simulink model "mdl4_20160413_004644"  (R2014a)
settings: Solver=FixedStepDiscrete  SolverMode=SingleTasking  StartTime=TIME(1)  StopTime=TIME(end)  FixedStep=SIMSTEP  RelTol=1e-3
model workspace (MAT data in the model file):
  autoc_mdd_data01 : struct (value not decoded)
undefined symbols (not defined in the file): Parameter113, Parameter131, Parameter132, Parameter144, Parameter51, Parameter52, Parameter53, Parameter54, Parameter69, Parameter91, SIMSTEP
(part 3 of 3)

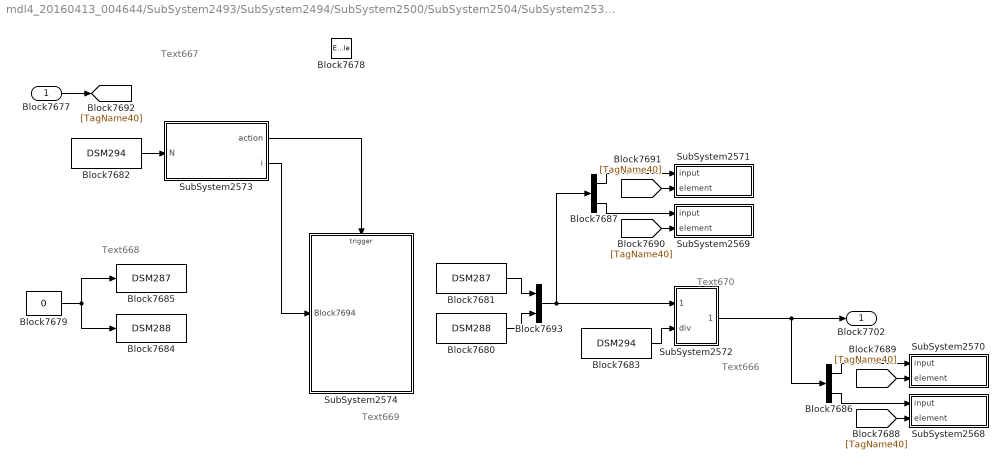
== system mdl4_20160413_004644/SubSystem2493/SubSystem2494/SubSystem2500/SubSystem2504/SubSystem2533/SubSystem2567 ==
  note: Text670
  note: Text669
  note: Text668
  note: Text667
  note: Text666
  Block7677 : Inport
  Block7678 : EnablePort
  Block7679 : Constant  Value=0  OutDataTypeStr=double  SampleTime=-1
  Block7680 : DataStoreRead  Priority=30  DataStoreName=DSM288
      settings: AttributesFormatString=Attribute1963
  Block7681 : DataStoreRead  Priority=30  DataStoreName=DSM287
      settings: AttributesFormatString=Attribute1964
  Block7682 : DataStoreRead  DataStoreName=DSM294
  Block7683 : DataStoreRead  DataStoreName=DSM294
  Block7684 : DataStoreWrite  Priority=10  DataStoreName=DSM288
      settings: AttributesFormatString=Attribute1965
  Block7685 : DataStoreWrite  Priority=10  DataStoreName=DSM287
      settings: AttributesFormatString=Attribute1966
  Block7686 : Demux  Outputs=2
  Block7687 : Demux  Outputs=2
  Block7693 : Mux  Inputs=2
  SubSystem2568 : Subsystem  TreatAsAtomicUnit=on  mask(***ATC.DSWVEC***){bd_version=1.01.A, r0=DSM290, r1=-1, r2=, r3=, r4=, r5=, r6=, r7=, r8=, r9=, c0=, c1=, c2=, c3=, c4=, c5=, c6=, c7=, c8=, c9=}
      mask prompts: bd_version "Version"
      mask help: これはAutoCからのブロックです．編集禁止．
      settings: OpenFcn=warndlg('変更禁止!');
      mask Help: web(ui_blockhelpmng(gcb));
      mask Display: disp('ATC.DSRVEC')
  SubSystem2569 : Subsystem  TreatAsAtomicUnit=on  mask(***ATC.DSWVEC***){bd_version=1.01.A, r0=DSM292, r1=-1, r2=, r3=, r4=, r5=, r6=, r7=, r8=, r9=, c0=, c1=, c2=, c3=, c4=, c5=, c6=, c7=, c8=, c9=}
      mask prompts: bd_version "Version"
      mask help: これはAutoCからのブロックです．編集禁止．
      settings: OpenFcn=warndlg('変更禁止!');
      mask Help: web(ui_blockhelpmng(gcb));
      mask Display: disp('ATC.DSRVEC')
  SubSystem2570 : Subsystem  TreatAsAtomicUnit=on  mask(***ATC.DSWVEC***){bd_version=1.01.A, r0=DSM289, r1=-1, r2=, r3=, r4=, r5=, r6=, r7=, r8=, r9=, c0=, c1=, c2=, c3=, c4=, c5=, c6=, c7=, c8=, c9=}
      mask prompts: bd_version "Version"
      mask help: これはAutoCからのブロックです．編集禁止．
      settings: OpenFcn=warndlg('変更禁止!');
      mask Help: web(ui_blockhelpmng(gcb));
      mask Display: disp('ATC.DSRVEC')
  SubSystem2571 : Subsystem  TreatAsAtomicUnit=on  mask(***ATC.DSWVEC***){bd_version=1.01.A, r0=DSM291, r1=-1, r2=, r3=, r4=, r5=, r6=, r7=, r8=, r9=, c0=, c1=, c2=, c3=, c4=, c5=, c6=, c7=, c8=, c9=}
      mask prompts: bd_version "Version"
      mask help: これはAutoCからのブロックです．編集禁止．
      settings: OpenFcn=warndlg('変更禁止!');
      mask Help: web(ui_blockhelpmng(gcb));
      mask Display: disp('ATC.DSRVEC')
  SubSystem2572 : Subsystem  TreatAsAtomicUnit=on  mask(***ATC.DIVISION***){bd_version=1.01.A, r0=チェック無し, r1=, r2=, r3=, r4=, r5=, r6=, r7=, r8=, r9=, c0=, c1=, c2=, c3=, c4=, c5=, c6=, c7=, c8=, c9=}
      mask prompts: bd_version "Version"
      mask help: これはAutoCからのブロックです．編集禁止．
      settings: OpenFcn=warndlg('変更禁止!');
      mask Help: web(ui_blockhelpmng(gcb));
  SubSystem2573 : Subsystem  Priority=20  TreatAsAtomicUnit=on  mask(***ATC.ITERATOR***){}
      mask help: これはAutoCからのブロックです．編集禁止．
      settings: AttributesFormatString=Attribute1967  OpenFcn=warndlg('変更禁止!');  RTWSystemCode=Inline
  SubSystem2574 : Subsystem  TreatAsAtomicUnit=on
  Block7702 : Outport
  wires:
  Block7679/1 -> Block7684/1, Block7685/1
  Block7687/2 -> SubSystem2569/1(input)
  [TagName40] -> SubSystem2569/2(element)
  Block7687/1 -> SubSystem2571/1(input)
  [TagName40] -> SubSystem2571/2(element)
  Block7686/2 -> SubSystem2568/1(input)
  [TagName40] -> SubSystem2568/2(element)
  Block7686/1 -> SubSystem2570/1(input)
  [TagName40] -> SubSystem2570/2(element)
  Block7693/1 -> Block7687/1, SubSystem2572/1(mult)
  Block7680/1 -> Block7693/2
  Block7681/1 -> Block7693/1
  SubSystem2572/1(Out) -> Block7686/1, Block7702/1
  Block7683/1 -> SubSystem2572/2(div)
  SubSystem2573/2(i) -> SubSystem2574/1(Block7694)
  SubSystem2573/1(action) -> SubSystem2574/Trigger
  Block7682/1 -> SubSystem2573/1(N)
  Block7677/1 -> [TagName40]

== system mdl4_20160413_004644/SubSystem2493/SubSystem2494/SubSystem2500/SubSystem2504/SubSystem2533/SubSystem2537/SubSystem2538 ==
  note: ***編集禁止***
  input : Inport
  element : Inport  Port=2
  Assignment : Assignment  IndexOptions=Index vector (port)  OutputSizes=[1 1]
  Inside_DSR : DataStoreRead  DataStoreName=DSM293
  Inside_DSW : DataStoreWrite  DataStoreName=DSM293
  wires:
  Assignment/1 -> Inside_DSW/1
  Inside_DSR/1 -> Assignment/1
  input/1 -> Assignment/2
  element/1 -> Assignment/3

== system mdl4_20160413_004644/SubSystem2493/SubSystem2494/SubSystem2500/SubSystem2504/SubSystem2533/SubSystem2537/SubSystem2539 ==
  note: ***編集禁止***
  input : Inport
  element : Inport  Port=2
  Assignment : Assignment  IndexOptions=Index vector (port)  OutputSizes=[1 1]
  Inside_DSR : DataStoreRead  DataStoreName=DSM295
  Inside_DSW : DataStoreWrite  DataStoreName=DSM295
  wires:
  Assignment/1 -> Inside_DSW/1
  Inside_DSR/1 -> Assignment/1
  input/1 -> Assignment/2
  element/1 -> Assignment/3

== system mdl4_20160413_004644/SubSystem2493/SubSystem2494/SubSystem2500/SubSystem2504/SubSystem2533/SubSystem2537/SubSystem2540 ==
  note: ***編集禁止***
  In1 : Inport
  In2 : Inport  Port=2
  RO1 : RelationalOperator  Operator===  InputSameDT=on
  single1 : DataTypeConversion  OutDataTypeStr=single  SaturateOnIntegerOverflow=on  RndMeth=Zero
  single2 : DataTypeConversion  OutDataTypeStr=single  SaturateOnIntegerOverflow=on  RndMeth=Zero
  Out1 : Outport
  wires:
  single2/1 -> RO1/2
  single1/1 -> RO1/1
  In1/1 -> single1/1
  In2/1 -> single2/1
  RO1/1 -> Out1/1

== system mdl4_20160413_004644/SubSystem2493/SubSystem2494/SubSystem2500/SubSystem2504/SubSystem2533/SubSystem2541/SubSystem2542 ==
  note: ***編集禁止***
  input : Inport
  element : Inport  Port=2
  Assignment : Assignment  IndexOptions=Index vector (port)  OutputSizes=[1 1]
  Inside_DSR : DataStoreRead  DataStoreName=DSM279
  Inside_DSW : DataStoreWrite  DataStoreName=DSM279
  wires:
  Assignment/1 -> Inside_DSW/1
  Inside_DSR/1 -> Assignment/1
  input/1 -> Assignment/2
  element/1 -> Assignment/3

== system mdl4_20160413_004644/SubSystem2493/SubSystem2494/SubSystem2500/SubSystem2504/SubSystem2533/SubSystem2541/SubSystem2543 ==
  note: ***編集禁止***
  input : Inport
  element : Inport  Port=2
  Assignment : Assignment  IndexOptions=Index vector (port)  OutputSizes=[1 1]
  Inside_DSR : DataStoreRead  DataStoreName=DSM280
  Inside_DSW : DataStoreWrite  DataStoreName=DSM280
  wires:
  Assignment/1 -> Inside_DSW/1
  Inside_DSR/1 -> Assignment/1
  input/1 -> Assignment/2
  element/1 -> Assignment/3

== system mdl4_20160413_004644/SubSystem2493/SubSystem2494/SubSystem2500/SubSystem2504/SubSystem2533/SubSystem2544/SubSystem2545 ==
  note: ***編集禁止***
  input : Inport
  element : Inport  Port=2
  Assignment : Assignment  IndexOptions=Index vector (port)  OutputSizes=[1 1]
  Inside_DSR : DataStoreRead  DataStoreName=DSM281
  Inside_DSW : DataStoreWrite  DataStoreName=DSM281
  wires:
  Assignment/1 -> Inside_DSW/1
  Inside_DSR/1 -> Assignment/1
  input/1 -> Assignment/2
  element/1 -> Assignment/3

== system mdl4_20160413_004644/SubSystem2493/SubSystem2494/SubSystem2500/SubSystem2504/SubSystem2533/SubSystem2544/SubSystem2546 ==
  note: ***編集禁止***
  input : Inport
  element : Inport  Port=2
  Assignment : Assignment  IndexOptions=Index vector (port)  OutputSizes=[1 1]
  Inside_DSR : DataStoreRead  DataStoreName=DSM282
  Inside_DSW : DataStoreWrite  DataStoreName=DSM282
  wires:
  Assignment/1 -> Inside_DSW/1
  Inside_DSR/1 -> Assignment/1
  input/1 -> Assignment/2
  element/1 -> Assignment/3

== system mdl4_20160413_004644/SubSystem2493/SubSystem2494/SubSystem2500/SubSystem2504/SubSystem2533/SubSystem2547/SubSystem2548 ==
  note: ***編集禁止***
  input : Inport
  element : Inport  Port=2
  Assignment : Assignment  IndexOptions=Index vector (port)  OutputSizes=[1 1]
  Inside_DSR : DataStoreRead  DataStoreName=DSM290
  Inside_DSW : DataStoreWrite  DataStoreName=DSM290
  wires:
  Assignment/1 -> Inside_DSW/1
  Inside_DSR/1 -> Assignment/1
  input/1 -> Assignment/2
  element/1 -> Assignment/3

== system mdl4_20160413_004644/SubSystem2493/SubSystem2494/SubSystem2500/SubSystem2504/SubSystem2533/SubSystem2547/SubSystem2549 ==
  note: ***編集禁止***
  input : Inport
  element : Inport  Port=2
  Assignment : Assignment  IndexOptions=Index vector (port)  OutputSizes=[1 1]
  Inside_DSR : DataStoreRead  DataStoreName=DSM292
  Inside_DSW : DataStoreWrite  DataStoreName=DSM292
  wires:
  element/1 -> Assignment/3
  input/1 -> Assignment/2
  Inside_DSR/1 -> Assignment/1
  Assignment/1 -> Inside_DSW/1

== system mdl4_20160413_004644/SubSystem2493/SubSystem2494/SubSystem2500/SubSystem2504/SubSystem2533/SubSystem2547/SubSystem2550 ==
  note: ***編集禁止***
  input : Inport
  element : Inport  Port=2
  Assignment : Assignment  IndexOptions=Index vector (port)  OutputSizes=[1 1]
  Inside_DSR : DataStoreRead  DataStoreName=DSM289
  Inside_DSW : DataStoreWrite  DataStoreName=DSM289
  wires:
  element/1 -> Assignment/3
  input/1 -> Assignment/2
  Inside_DSR/1 -> Assignment/1
  Assignment/1 -> Inside_DSW/1

== system mdl4_20160413_004644/SubSystem2493/SubSystem2494/SubSystem2500/SubSystem2504/SubSystem2533/SubSystem2547/SubSystem2551 ==
  note: ***編集禁止***
  input : Inport
  element : Inport  Port=2
  Assignment : Assignment  IndexOptions=Index vector (port)  OutputSizes=[1 1]
  Inside_DSR : DataStoreRead  DataStoreName=DSM291
  Inside_DSW : DataStoreWrite  DataStoreName=DSM291
  wires:
  Assignment/1 -> Inside_DSW/1
  Inside_DSR/1 -> Assignment/1
  input/1 -> Assignment/2
  element/1 -> Assignment/3

== system mdl4_20160413_004644/SubSystem2493/SubSystem2494/SubSystem2500/SubSystem2504/SubSystem2533/SubSystem2547/SubSystem2552 ==
  note: ***編集禁止***
  mult : Inport
  div : Inport  Port=2
  Product : Product  Inputs=*/  SaturateOnIntegerOverflow=on  RndMeth=Zero  InputSameDT=on  OutDataTypeStr=Inherit: Same as first input
  Out : Outport
  wires:
  Product/1 -> Out/1
  mult/1 -> Product/1
  div/1 -> Product/2

== system mdl4_20160413_004644/SubSystem2493/SubSystem2494/SubSystem2500/SubSystem2504/SubSystem2533/SubSystem2547/SubSystem2553 ==
  note: ***編集禁止***
  N : Inport
  For_loop : Stateflow chart  TreatAsAtomicUnit=on
  action : Outport
  i : Outport  Port=2
  wires:
  For_loop/1(idx) -> i/1
  N/1 -> For_loop/1(N_Loop)
  For_loop/2(function_call()) -> action/1

== system mdl4_20160413_004644/SubSystem2493/SubSystem2494/SubSystem2500/SubSystem2504/SubSystem2533/SubSystem2547/SubSystem2554 ==
  note: Text645
  note: Text644
  note: Text643
  note: Text642
  note: Text641
  Block7642 : Inport
  Block7643 : TriggerPort  TriggerType=function-call
  Block7644 : DataStoreRead  DataStoreName=DSM288
  Block7645 : DataStoreRead  DataStoreName=DSM287
  Block7646 : DataStoreWrite  DataStoreName=DSM288
  Block7647 : DataStoreWrite  DataStoreName=DSM287
  Block7648 : Sum  Inputs=++|  OutDataTypeStr=double  RndMeth=Zero  SaturateOnIntegerOverflow=on  InputSameDT=on
  Block7649 : Sum  Inputs=++|  OutDataTypeStr=double  RndMeth=Zero  SaturateOnIntegerOverflow=on  InputSameDT=on
  SubSystem2555 : Subsystem  TreatAsAtomicUnit=on  mask(***ATC.DSRVEC***){bd_version=1.01.A, r0=DSM293, r1=-1, r2=, r3=, r4=, r5=, r6=, r7=, r8=, r9=, c0=, c1=, c2=, c3=, c4=, c5=, c6=, c7=, c8=, c9=}
      mask prompts: bd_version "Version"
      mask help: これはAutoCからのブロックです．編集禁止．
      settings: OpenFcn=warndlg('変更禁止!');
      mask Help: web(ui_blockhelpmng(gcb));
      mask Display: disp('ATC.DSRVEC')
  SubSystem2556 : Subsystem  TreatAsAtomicUnit=on  mask(***ATC.DSRVEC***){bd_version=1.01.A, r0=DSM295, r1=-1, r2=, r3=, r4=, r5=, r6=, r7=, r8=, r9=, c0=, c1=, c2=, c3=, c4=, c5=, c6=, c7=, c8=, c9=}
      mask prompts: bd_version "Version"
      mask help: これはAutoCからのブロックです．編集禁止．
      settings: OpenFcn=warndlg('変更禁止!');
      mask Help: web(ui_blockhelpmng(gcb));
      mask Display: disp('ATC.DSRVEC')
  wires:
  Block7648/1 -> Block7646/1
  Block7644/1 -> Block7648/1
  Block7649/1 -> Block7647/1
  Block7645/1 -> Block7649/1
  SubSystem2555/1(Output) -> Block7649/2  "SigLabel295"
  Block7642/1 -> SubSystem2555/1(element), SubSystem2556/1(element)
  SubSystem2556/1(Output) -> Block7648/2  "SigLabel294"

== system mdl4_20160413_004644/SubSystem2493/SubSystem2494/SubSystem2500/SubSystem2504/SubSystem2533/SubSystem2557/SubSystem2558 ==
  note: ***編集禁止***
  input : Inport
  element : Inport  Port=2
  Assignment : Assignment  IndexOptions=Index vector (port)  OutputSizes=[1 1]
  Inside_DSR : DataStoreRead  DataStoreName=DSM290
  Inside_DSW : DataStoreWrite  DataStoreName=DSM290
  wires:
  element/1 -> Assignment/3
  input/1 -> Assignment/2
  Inside_DSR/1 -> Assignment/1
  Assignment/1 -> Inside_DSW/1

== system mdl4_20160413_004644/SubSystem2493/SubSystem2494/SubSystem2500/SubSystem2504/SubSystem2533/SubSystem2557/SubSystem2559 ==
  note: ***編集禁止***
  input : Inport
  element : Inport  Port=2
  Assignment : Assignment  IndexOptions=Index vector (port)  OutputSizes=[1 1]
  Inside_DSR : DataStoreRead  DataStoreName=DSM292
  Inside_DSW : DataStoreWrite  DataStoreName=DSM292
  wires:
  Assignment/1 -> Inside_DSW/1
  Inside_DSR/1 -> Assignment/1
  input/1 -> Assignment/2
  element/1 -> Assignment/3

== system mdl4_20160413_004644/SubSystem2493/SubSystem2494/SubSystem2500/SubSystem2504/SubSystem2533/SubSystem2557/SubSystem2560 ==
  note: ***編集禁止***
  input : Inport
  element : Inport  Port=2
  Assignment : Assignment  IndexOptions=Index vector (port)  OutputSizes=[1 1]
  Inside_DSR : DataStoreRead  DataStoreName=DSM289
  Inside_DSW : DataStoreWrite  DataStoreName=DSM289
  wires:
  Assignment/1 -> Inside_DSW/1
  Inside_DSR/1 -> Assignment/1
  input/1 -> Assignment/2
  element/1 -> Assignment/3

== system mdl4_20160413_004644/SubSystem2493/SubSystem2494/SubSystem2500/SubSystem2504/SubSystem2533/SubSystem2557/SubSystem2561 ==
  note: ***編集禁止***
  input : Inport
  element : Inport  Port=2
  Assignment : Assignment  IndexOptions=Index vector (port)  OutputSizes=[1 1]
  Inside_DSR : DataStoreRead  DataStoreName=DSM291
  Inside_DSW : DataStoreWrite  DataStoreName=DSM291
  wires:
  element/1 -> Assignment/3
  input/1 -> Assignment/2
  Inside_DSR/1 -> Assignment/1
  Assignment/1 -> Inside_DSW/1

== system mdl4_20160413_004644/SubSystem2493/SubSystem2494/SubSystem2500/SubSystem2504/SubSystem2533/SubSystem2557/SubSystem2562 ==
  note: ***編集禁止***
  mult : Inport
  div : Inport  Port=2
  Product : Product  Inputs=*/  SaturateOnIntegerOverflow=on  RndMeth=Zero  InputSameDT=on  OutDataTypeStr=Inherit: Same as first input
  Out : Outport
  wires:
  div/1 -> Product/2
  mult/1 -> Product/1
  Product/1 -> Out/1

== system mdl4_20160413_004644/SubSystem2493/SubSystem2494/SubSystem2500/SubSystem2504/SubSystem2533/SubSystem2557/SubSystem2563 ==
  note: ***編集禁止***
  N : Inport
  For_loop : Stateflow chart  TreatAsAtomicUnit=on
  action : Outport
  i : Outport  Port=2
  wires:
  For_loop/1(idx) -> i/1
  N/1 -> For_loop/1(N_Loop)
  For_loop/2(function_call()) -> action/1

== system mdl4_20160413_004644/SubSystem2493/SubSystem2494/SubSystem2500/SubSystem2504/SubSystem2533/SubSystem2557/SubSystem2564 ==
  note: Text655
  note: Text654
  note: Text653
  note: Text652
  note: Text651
  Block7668 : Inport
  Block7669 : TriggerPort  TriggerType=function-call
  Block7670 : DataStoreRead  DataStoreName=DSM288
  Block7671 : DataStoreRead  DataStoreName=DSM287
  Block7672 : DataStoreWrite  DataStoreName=DSM288
  Block7673 : DataStoreWrite  DataStoreName=DSM287
  Block7674 : Sum  Inputs=++|  OutDataTypeStr=double  RndMeth=Zero  SaturateOnIntegerOverflow=on  InputSameDT=on
  Block7675 : Sum  Inputs=++|  OutDataTypeStr=double  RndMeth=Zero  SaturateOnIntegerOverflow=on  InputSameDT=on
  SubSystem2565 : Subsystem  TreatAsAtomicUnit=on  mask(***ATC.DSRVEC***){bd_version=1.01.A, r0=DSM279, r1=-1, r2=, r3=, r4=, r5=, r6=, r7=, r8=, r9=, c0=, c1=, c2=, c3=, c4=, c5=, c6=, c7=, c8=, c9=}
      mask prompts: bd_version "Version"
      mask help: これはAutoCからのブロックです．編集禁止．
      settings: OpenFcn=warndlg('変更禁止!');
      mask Help: web(ui_blockhelpmng(gcb));
      mask Display: disp('ATC.DSRVEC')
  SubSystem2566 : Subsystem  TreatAsAtomicUnit=on  mask(***ATC.DSRVEC***){bd_version=1.01.A, r0=DSM280, r1=-1, r2=, r3=, r4=, r5=, r6=, r7=, r8=, r9=, c0=, c1=, c2=, c3=, c4=, c5=, c6=, c7=, c8=, c9=}
      mask prompts: bd_version "Version"
      mask help: これはAutoCからのブロックです．編集禁止．
      settings: OpenFcn=warndlg('変更禁止!');
      mask Help: web(ui_blockhelpmng(gcb));
      mask Display: disp('ATC.DSRVEC')
  wires:
  SubSystem2566/1(Output) -> Block7674/2  "SigLabel297"
  Block7668/1 -> SubSystem2565/1(element), SubSystem2566/1(element)
  SubSystem2565/1(Output) -> Block7675/2  "SigLabel296"
  Block7671/1 -> Block7675/1
  Block7675/1 -> Block7673/1
  Block7670/1 -> Block7674/1
  Block7674/1 -> Block7672/1

== system mdl4_20160413_004644/SubSystem2493/SubSystem2494/SubSystem2500/SubSystem2504/SubSystem2533/SubSystem2567/SubSystem2568 ==
  note: ***編集禁止***
  input : Inport
  element : Inport  Port=2
  Assignment : Assignment  IndexOptions=Index vector (port)  OutputSizes=[1 1]
  Inside_DSR : DataStoreRead  DataStoreName=DSM290
  Inside_DSW : DataStoreWrite  DataStoreName=DSM290
  wires:
  Assignment/1 -> Inside_DSW/1
  Inside_DSR/1 -> Assignment/1
  input/1 -> Assignment/2
  element/1 -> Assignment/3

== system mdl4_20160413_004644/SubSystem2493/SubSystem2494/SubSystem2500/SubSystem2504/SubSystem2533/SubSystem2567/SubSystem2569 ==
  note: ***編集禁止***
  input : Inport
  element : Inport  Port=2
  Assignment : Assignment  IndexOptions=Index vector (port)  OutputSizes=[1 1]
  Inside_DSR : DataStoreRead  DataStoreName=DSM292
  Inside_DSW : DataStoreWrite  DataStoreName=DSM292
  wires:
  element/1 -> Assignment/3
  input/1 -> Assignment/2
  Inside_DSR/1 -> Assignment/1
  Assignment/1 -> Inside_DSW/1

== system mdl4_20160413_004644/SubSystem2493/SubSystem2494/SubSystem2500/SubSystem2504/SubSystem2533/SubSystem2567/SubSystem2570 ==
  note: ***編集禁止***
  input : Inport
  element : Inport  Port=2
  Assignment : Assignment  IndexOptions=Index vector (port)  OutputSizes=[1 1]
  Inside_DSR : DataStoreRead  DataStoreName=DSM289
  Inside_DSW : DataStoreWrite  DataStoreName=DSM289
  wires:
  element/1 -> Assignment/3
  input/1 -> Assignment/2
  Inside_DSR/1 -> Assignment/1
  Assignment/1 -> Inside_DSW/1

== system mdl4_20160413_004644/SubSystem2493/SubSystem2494/SubSystem2500/SubSystem2504/SubSystem2533/SubSystem2567/SubSystem2571 ==
  note: ***編集禁止***
  input : Inport
  element : Inport  Port=2
  Assignment : Assignment  IndexOptions=Index vector (port)  OutputSizes=[1 1]
  Inside_DSR : DataStoreRead  DataStoreName=DSM291
  Inside_DSW : DataStoreWrite  DataStoreName=DSM291
  wires:
  Assignment/1 -> Inside_DSW/1
  Inside_DSR/1 -> Assignment/1
  input/1 -> Assignment/2
  element/1 -> Assignment/3

== system mdl4_20160413_004644/SubSystem2493/SubSystem2494/SubSystem2500/SubSystem2504/SubSystem2533/SubSystem2567/SubSystem2572 ==
  note: ***編集禁止***
  mult : Inport
  div : Inport  Port=2
  Product : Product  Inputs=*/  SaturateOnIntegerOverflow=on  RndMeth=Zero  InputSameDT=on  OutDataTypeStr=Inherit: Same as first input
  Out : Outport
  wires:
  Product/1 -> Out/1
  mult/1 -> Product/1
  div/1 -> Product/2

== system mdl4_20160413_004644/SubSystem2493/SubSystem2494/SubSystem2500/SubSystem2504/SubSystem2533/SubSystem2567/SubSystem2573 ==
  note: ***編集禁止***
  N : Inport
  For_loop : Stateflow chart  TreatAsAtomicUnit=on
  action : Outport
  i : Outport  Port=2
  wires:
  For_loop/1(idx) -> i/1
  N/1 -> For_loop/1(N_Loop)
  For_loop/2(function_call()) -> action/1

== system mdl4_20160413_004644/SubSystem2493/SubSystem2494/SubSystem2500/SubSystem2504/SubSystem2533/SubSystem2567/SubSystem2574 ==
  note: Text665
  note: Text664
  note: Text663
  note: Text662
  note: Text661
  Block7694 : Inport
  Block7695 : TriggerPort  TriggerType=function-call
  Block7696 : DataStoreRead  DataStoreName=DSM288
  Block7697 : DataStoreRead  DataStoreName=DSM287
  Block7698 : DataStoreWrite  DataStoreName=DSM288
  Block7699 : DataStoreWrite  DataStoreName=DSM287
  Block7700 : Sum  Inputs=++|  OutDataTypeStr=double  RndMeth=Zero  SaturateOnIntegerOverflow=on  InputSameDT=on
  Block7701 : Sum  Inputs=++|  OutDataTypeStr=double  RndMeth=Zero  SaturateOnIntegerOverflow=on  InputSameDT=on
  SubSystem2575 : Subsystem  TreatAsAtomicUnit=on  mask(***ATC.DSRVEC***){bd_version=1.01.A, r0=DSM281, r1=-1, r2=, r3=, r4=, r5=, r6=, r7=, r8=, r9=, c0=, c1=, c2=, c3=, c4=, c5=, c6=, c7=, c8=, c9=}
      mask prompts: bd_version "Version"
      mask help: これはAutoCからのブロックです．編集禁止．
      settings: OpenFcn=warndlg('変更禁止!');
      mask Help: web(ui_blockhelpmng(gcb));
      mask Display: disp('ATC.DSRVEC')
  SubSystem2576 : Subsystem  TreatAsAtomicUnit=on  mask(***ATC.DSRVEC***){bd_version=1.01.A, r0=DSM282, r1=-1, r2=, r3=, r4=, r5=, r6=, r7=, r8=, r9=, c0=, c1=, c2=, c3=, c4=, c5=, c6=, c7=, c8=, c9=}
      mask prompts: bd_version "Version"
      mask help: これはAutoCからのブロックです．編集禁止．
      settings: OpenFcn=warndlg('変更禁止!');
      mask Help: web(ui_blockhelpmng(gcb));
      mask Display: disp('ATC.DSRVEC')
  wires:
  Block7700/1 -> Block7698/1
  Block7696/1 -> Block7700/1
  Block7701/1 -> Block7699/1
  Block7697/1 -> Block7701/1
  SubSystem2575/1(Output) -> Block7701/2  "SigLabel299"
  Block7694/1 -> SubSystem2575/1(element), SubSystem2576/1(element)
  SubSystem2576/1(Output) -> Block7700/2  "SigLabel298"

== system mdl4_20160413_004644/SubSystem2493/SubSystem2494/SubSystem2500/SubSystem2504/SubSystem2533/SubSystem2547/SubSystem2554/SubSystem2555 ==
  note: ***編集禁止***
  element : Inport
  Inside_DSR : DataStoreRead  DataStoreName=DSM293
  Selector : Selector  IndexOptions=Index vector (port)  Indices=[1 3]
  Output : Outport
  wires:
  Inside_DSR/1 -> Selector/1
  element/1 -> Selector/2
  Selector/1 -> Output/1

== system mdl4_20160413_004644/SubSystem2493/SubSystem2494/SubSystem2500/SubSystem2504/SubSystem2533/SubSystem2547/SubSystem2554/SubSystem2556 ==
  note: ***編集禁止***
  element : Inport
  Inside_DSR : DataStoreRead  DataStoreName=DSM295
  Selector : Selector  IndexOptions=Index vector (port)  Indices=[1 3]
  Output : Outport
  wires:
  Selector/1 -> Output/1
  element/1 -> Selector/2
  Inside_DSR/1 -> Selector/1

== system mdl4_20160413_004644/SubSystem2493/SubSystem2494/SubSystem2500/SubSystem2504/SubSystem2533/SubSystem2557/SubSystem2564/SubSystem2565 ==
  note: ***編集禁止***
  element : Inport
  Inside_DSR : DataStoreRead  DataStoreName=DSM279
  Selector : Selector  IndexOptions=Index vector (port)  Indices=[1 3]
  Output : Outport
  wires:
  Inside_DSR/1 -> Selector/1
  element/1 -> Selector/2
  Selector/1 -> Output/1

== system mdl4_20160413_004644/SubSystem2493/SubSystem2494/SubSystem2500/SubSystem2504/SubSystem2533/SubSystem2557/SubSystem2564/SubSystem2566 ==
  note: ***編集禁止***
  element : Inport
  Inside_DSR : DataStoreRead  DataStoreName=DSM280
  Selector : Selector  IndexOptions=Index vector (port)  Indices=[1 3]
  Output : Outport
  wires:
  Selector/1 -> Output/1
  element/1 -> Selector/2
  Inside_DSR/1 -> Selector/1

== system mdl4_20160413_004644/SubSystem2493/SubSystem2494/SubSystem2500/SubSystem2504/SubSystem2533/SubSystem2567/SubSystem2574/SubSystem2575 ==
  note: ***編集禁止***
  element : Inport
  Inside_DSR : DataStoreRead  DataStoreName=DSM281
  Selector : Selector  IndexOptions=Index vector (port)  Indices=[1 3]
  Output : Outport
  wires:
  Inside_DSR/1 -> Selector/1
  element/1 -> Selector/2
  Selector/1 -> Output/1

== system mdl4_20160413_004644/SubSystem2493/SubSystem2494/SubSystem2500/SubSystem2504/SubSystem2533/SubSystem2567/SubSystem2574/SubSystem2576 ==
  note: ***編集禁止***
  element : Inport
  Inside_DSR : DataStoreRead  DataStoreName=DSM282
  Selector : Selector  IndexOptions=Index vector (port)  Indices=[1 3]
  Output : Outport
  wires:
  Selector/1 -> Output/1
  element/1 -> Selector/2
  Inside_DSR/1 -> Selector/1

== stateflow chart mdl4_20160413_004644/SubSystem2493/SubSystem2494/SubSystem2500/SubSystem2504/SubSystem2533/SubSystem2557/SubSystem2563/For_loop ==
  note: for(i1 = 0; i1 < N_Loop; i1++) {
      |   処理
      | }
  (default) -> (junction 8) : {
      |  idx = 1;
      |  i1 = 0;
      | }
  (junction 11) -> (junction 8) : {i1++;}
  (junction 8) -> (junction 9)
  (junction 10) -> (junction 11) : {
      |  function_call;
      |  idx = idx + 1;
      | }
  (junction 9) -> (junction 10) [order 1] : [i1 < N_Loop]
  (junction 9) -> (junction 12) [order 2]
  data: N_Loop input; i1 local int32; idx output
  events: function_call output FUNCTION_CALL_EVENT

== stateflow chart mdl4_20160413_004644/SubSystem2493/SubSystem2494/SubSystem2500/SubSystem2504/SubSystem2533/SubSystem2547/SubSystem2553/For_loop ==
  note: for(i1 = 0; i1 < N_Loop; i1++) {
      |   処理
      | }
  (default) -> (junction 8) : {
      |  idx = 1;
      |  i1 = 0;
      | }
  (junction 11) -> (junction 8) : {i1++;}
  (junction 8) -> (junction 9)
  (junction 10) -> (junction 11) : {
      |  function_call;
      |  idx = idx + 1;
      | }
  (junction 9) -> (junction 10) [order 1] : [i1 < N_Loop]
  (junction 9) -> (junction 12) [order 2]
  data: N_Loop input; i1 local int32; idx output
  events: function_call output FUNCTION_CALL_EVENT

== stateflow chart mdl4_20160413_004644/SubSystem2493/SubSystem2494/SubSystem2500/SubSystem2504/SubSystem2533/SubSystem2567/SubSystem2573/For_loop ==
  note: for(i1 = 0; i1 < N_Loop; i1++) {
      |   処理
      | }
  (default) -> (junction 8) : {
      |  idx = 1;
      |  i1 = 0;
      | }
  (junction 11) -> (junction 8) : {i1++;}
  (junction 8) -> (junction 9)
  (junction 10) -> (junction 11) : {
      |  function_call;
      |  idx = idx + 1;
      | }
  (junction 9) -> (junction 10) [order 1] : [i1 < N_Loop]
  (junction 9) -> (junction 12) [order 2]
  data: N_Loop input; i1 local int32; idx output
  events: function_call output FUNCTION_CALL_EVENT

== stateflow chart mdl4_20160413_004644/SubSystem2493/SubSystem2577/SubSystem2579/SubSystem2580/For_loop ==
  note: for(i1 = 0; i1 < N_Loop; i1++) {
      |   処理
      | }
  (default) -> (junction 8) : {
      |  idx = 1;
      |  i1 = 0;
      | }
  (junction 11) -> (junction 8) : {i1++;}
  (junction 8) -> (junction 9)
  (junction 10) -> (junction 11) : {
      |  function_call;
      |  idx = idx + 1;
      | }
  (junction 9) -> (junction 10) [order 1] : [i1 < N_Loop]
  (junction 9) -> (junction 12) [order 2]
  data: N_Loop input; i1 local int32; idx output
  events: function_call output FUNCTION_CALL_EVENT
